simulink model "modelo"  (R2021b)
settings: Solver=VariableStepAuto  StartTime=0.0  StopTime=10.0  RelTol=1e-3
settings Model: Creator=iguil  LastModifiedBy=David

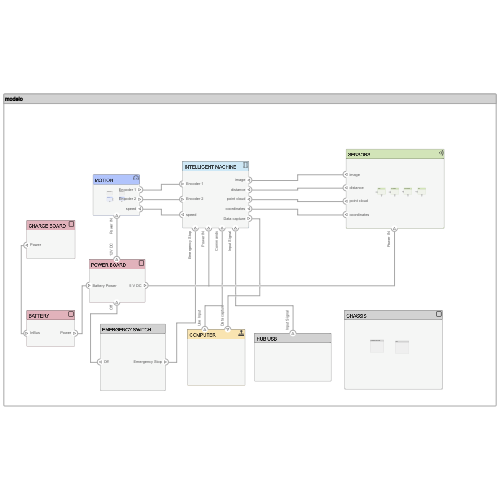
[thumbnail: Simulink's stored preview of the top-level diagram]
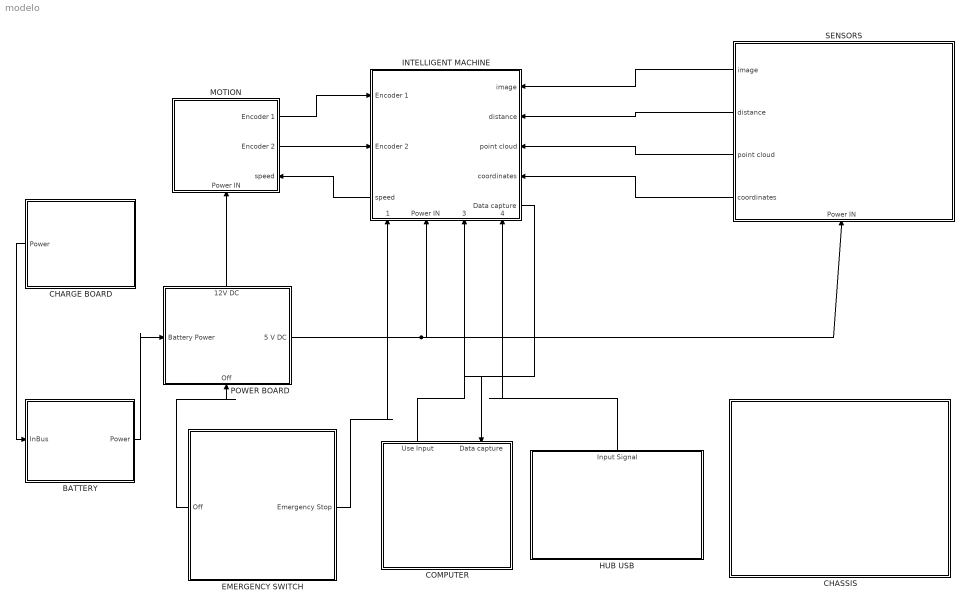
== system modelo ==
  BATTERY : Subsystem
      settings: PortSchema="{\"entries\":[{\"content\":{\"headerSize\":26,\"margin\":15,\"minimumSpacing\":25,\"sides\":[{\"content\":{\"connectorIds\":[\"In1\"]},\"type\":\"ConnectorPlacement.EquallySpacedRectSide\",\"uuid\":\"78ec9596-c19b-4a19-90cc-d79d904dcecb\"},{\"content\":{\"connectorIds\":[\"Out1\"],\"side\":\"RIGHT\"},\"type\":\"ConnectorPlacement.EquallySpacedRectSide\",\"uuid\":\"e50c32f8-61a1-4c3e-810e-7c092ec61b9d\"},{\"content\":{\"connectorIds\":[],\"side\":\"TOP\"},\"type\":\"ConnectorPlacement.EquallySpacedRectSide\",\"uuid\":\"dd5589de-c446-44bc-b6c3-43d178c94f81\"}]},\"type\":\"ConnectorPlacement.EquallySpacedConnector\",\"uuid\":\"1e9f716a-1f22-4423-b94e-8264810d47f5\"}],\"packageUris\":[\"http://schema.mathworks.com/mf0/Connector/R2020b\"],\"version\":\"1.0\"}"
  CHARGE BOARD : Subsystem
      settings: PortSchema="{\"entries\":[{\"content\":{\"headerSize\":26,\"margin\":15,\"minimumSpacing\":25,\"sides\":[{\"content\":{\"connectorIds\":[\"Out1\"]},\"type\":\"ConnectorPlacement.EquallySpacedRectSide\",\"uuid\":\"78ec9596-c19b-4a19-90cc-d79d904dcecb\"},{\"content\":{\"connectorIds\":[],\"side\":\"RIGHT\"},\"type\":\"ConnectorPlacement.EquallySpacedRectSide\",\"uuid\":\"e50c32f8-61a1-4c3e-810e-7c092ec61b9d\"},{\"content\":{\"connectorIds\":[],\"side\":\"TOP\"},\"type\":\"ConnectorPlacement.EquallySpacedRectSide\",\"uuid\":\"dd5589de-c446-44bc-b6c3-43d178c94f81\"},{\"content\":{\"connectorIds\":[],\"side\":\"BOTTOM\"},\"type\":\"ConnectorPlacement.EquallySpacedRectSide\",\"uuid\":\"27b2c156-9ba5-4a85-9e63-882de663826b\"}]},\"type\":\"ConnectorPlacement.EquallySpacedConnector\",\"uuid\":\"1e9f716a-1f22-4423-b94e-8264810d47f5\"}],\"packageUris\":[\"http://schema.mathworks.com/mf0/Connector/R2020b\"],\"version\":\"1.0\"}"
  CHASSIS : Subsystem
      settings: PortSchema="{\"entries\":[{\"content\":{\"headerSize\":26,\"margin\":15,\"minimumSpacing\":25,\"sides\":[{\"content\":{\"connectorIds\":[]},\"type\":\"ConnectorPlacement.EquallySpacedRectSide\",\"uuid\":\"78ec9596-c19b-4a19-90cc-d79d904dcecb\"},{\"content\":{\"connectorIds\":[],\"side\":\"RIGHT\"},\"type\":\"ConnectorPlacement.EquallySpacedRectSide\",\"uuid\":\"e50c32f8-61a1-4c3e-810e-7c092ec61b9d\"},{\"content\":{\"connectorIds\":[],\"side\":\"TOP\"},\"type\":\"ConnectorPlacement.EquallySpacedRectSide\",\"uuid\":\"dd5589de-c446-44bc-b6c3-43d178c94f81\"}]},\"type\":\"ConnectorPlacement.EquallySpacedConnector\",\"uuid\":\"1e9f716a-1f22-4423-b94e-8264810d47f5\"}],\"packageUris\":[\"http://schema.mathworks.com/mf0/Connector/R2020b\"],\"version\":\"1.0\"}"
  COMPUTER : Subsystem
      settings: PortSchema="{\"entries\":[{\"content\":{\"headerSize\":26,\"margin\":15,\"minimumSpacing\":25,\"sides\":[{\"content\":{\"connectorIds\":[]},\"type\":\"ConnectorPlacement.EquallySpacedRectSide\",\"uuid\":\"78ec9596-c19b-4a19-90cc-d79d904dcecb\"},{\"content\":{\"connectorIds\":[],\"side\":\"RIGHT\"},\"type\":\"ConnectorPlacement.EquallySpacedRectSide\",\"uuid\":\"e50c32f8-61a1-4c3e-810e-7c092ec61b9d\"},{\"content\":{\"connectorIds\":[\"Out1\",\"In1\"],\"side\":\"TOP\"},\"type\":\"ConnectorPlacement.EquallySpacedRectSide\",\"uuid\":\"dd5589de-c446-44bc-b6c3-43d178c94f81\"}]},\"type\":\"ConnectorPlacement.EquallySpacedConnector\",\"uuid\":\"1e9f716a-1f22-4423-b94e-8264810d47f5\"}],\"packageUris\":[\"http://schema.mathworks.com/mf0/Connector/R2020b\"],\"version\":\"1.0\"}"
  EMERGENCY SWITCH : Subsystem
      settings: PortSchema="{\"entries\":[{\"content\":{\"headerSize\":26,\"margin\":15,\"minimumSpacing\":25,\"sides\":[{\"content\":{\"connectorIds\":[\"Out1\"]},\"type\":\"ConnectorPlacement.EquallySpacedRectSide\",\"uuid\":\"b3e59be9-c011-4959-aae7-924c85fec7bb\"},{\"content\":{\"connectorIds\":[\"Out2\"],\"side\":\"RIGHT\"},\"type\":\"ConnectorPlacement.EquallySpacedRectSide\",\"uuid\":\"1b4348cb-da5a-4ff5-ba36-0dfb750bb370\"},{\"content\":{\"connectorIds\":[],\"side\":\"TOP\"},\"type\":\"ConnectorPlacement.EquallySpacedRectSide\",\"uuid\":\"b059a036-e728-494e-885b-23330087d2f9\"},{\"content\":{\"connectorIds\":[],\"side\":\"BOTTOM\"},\"type\":\"ConnectorPlacement.EquallySpacedRectSide\",\"uuid\":\"1d25428c-8dbd-4571-8b86-c34d6589503b\"}]},\"type\":\"ConnectorPlacement.EquallySpacedConnector\",\"uuid\":\"d162fe16-67ad-48b8-8b82-50f283e6c9c2\"}],\"packageUris\":[\"http://schema.mathworks.com/mf0/Connector/R2020b\"],\"version\":\"1.0\"}"
  HUB USB : Subsystem
      settings: PortSchema="{\"entries\":[{\"content\":{\"headerSize\":26,\"margin\":15,\"minimumSpacing\":25,\"sides\":[{\"content\":{\"connectorIds\":[]},\"type\":\"ConnectorPlacement.EquallySpacedRectSide\",\"uuid\":\"78ec9596-c19b-4a19-90cc-d79d904dcecb\"},{\"content\":{\"connectorIds\":[],\"side\":\"RIGHT\"},\"type\":\"ConnectorPlacement.EquallySpacedRectSide\",\"uuid\":\"e50c32f8-61a1-4c3e-810e-7c092ec61b9d\"},{\"content\":{\"connectorIds\":[\"Out1\"],\"side\":\"TOP\"},\"type\":\"ConnectorPlacement.EquallySpacedRectSide\",\"uuid\":\"dd5589de-c446-44bc-b6c3-43d178c94f81\"}]},\"type\":\"ConnectorPlacement.EquallySpacedConnector\",\"uuid\":\"1e9f716a-1f22-4423-b94e-8264810d47f5\"}],\"packageUris\":[\"http://schema.mathworks.com/mf0/Connector/R2020b\"],\"version\":\"1.0\"}"
  INTELLIGENT MACHINE : Subsystem
      settings: PortSchema="{\"entries\":[{\"content\":{\"headerSize\":26,\"margin\":15,\"minimumSpacing\":25,\"sides\":[{\"content\":{\"connectorIds\":[\"In8\",\"In9\",\"Out2\"]},\"type\":\"ConnectorPlacement.EquallySpacedRectSide\",\"uuid\":\"b3e59be9-c011-4959-aae7-924c85fec7bb\"},{\"content\":{\"connectorIds\":[\"In2\",\"In5\",\"In6\",\"In7\",\"Out1\"],\"side\":\"RIGHT\"},\"type\":\"ConnectorPlacement.EquallySpacedRectSide\",\"uuid\":\"1b4348cb-da5a-4ff5-ba36-0dfb750bb370\"},{\"content\":{\"connectorIds\":[],\"side\":\"TOP\"},\"type\":\"ConnectorPlacement.EquallySpacedRectSide\",\"uuid\":\"b059a036-e728-494e-885b-23330087d2f9\"},{\"content\":{\"connectorIds\":[\"In1\",\"In10\",\"In3\",\"In4\"],\"side\":\"BOTTOM\"},\"type\":\"ConnectorPlacement.EquallySpacedRectSide\",\"uuid\":\"1d25428c-8dbd-4571-8b86-c34d6589503b\"}]},\"type\":\"ConnectorPlacement.EquallySpacedConnector\",\"uuid\":\"d162fe16-67ad-48b8-8b82-50f283e6c9c2\"}],\"packageUris\":[\"http://schema.mathworks.com/mf0/Connector/R2020b\"],\"version\":\"1.0\"}"
  MOTION : Subsystem
      settings: PortSchema="{\"entries\":[{\"content\":{\"headerSize\":26,\"margin\":15,\"minimumSpacing\":25,\"sides\":[{\"content\":{\"connectorIds\":[]},\"type\":\"ConnectorPlacement.EquallySpacedRectSide\",\"uuid\":\"baaf5190-1ffc-4710-9f12-f4ddd1b73331\"},{\"content\":{\"connectorIds\":[\"Out1\",\"Out2\",\"In1\"],\"side\":\"RIGHT\"},\"type\":\"ConnectorPlacement.EquallySpacedRectSide\",\"uuid\":\"f5fb468f-cc96-476c-be3d-ed2ea869153e\"},{\"content\":{\"connectorIds\":[],\"side\":\"TOP\"},\"type\":\"ConnectorPlacement.EquallySpacedRectSide\",\"uuid\":\"45f5cb0d-60bf-4943-bb4c-a92d305a6805\"},{\"content\":{\"connectorIds\":[\"In2\"],\"side\":\"BOTTOM\"},\"type\":\"ConnectorPlacement.EquallySpacedRectSide\",\"uuid\":\"76d560be-4d0b-4cec-a6c5-6844847a893b\"}]},\"type\":\"ConnectorPlacement.EquallySpacedConnector\",\"uuid\":\"99c88219-ed2b-4820-8e38-f370b921e53e\"}],\"packageUris\":[\"http://schema.mathworks.com/mf0/Connector/R2020b\"],\"version\":\"1.0\"}"
  POWER BOARD : Subsystem
      settings: PortSchema="{\"entries\":[{\"content\":{\"headerSize\":26,\"margin\":15,\"minimumSpacing\":25,\"sides\":[{\"content\":{\"connectorIds\":[\"In2\"]},\"type\":\"ConnectorPlacement.EquallySpacedRectSide\",\"uuid\":\"baaf5190-1ffc-4710-9f12-f4ddd1b73331\"},{\"content\":{\"connectorIds\":[\"Out1\"],\"side\":\"RIGHT\"},\"type\":\"ConnectorPlacement.EquallySpacedRectSide\",\"uuid\":\"f5fb468f-cc96-476c-be3d-ed2ea869153e\"},{\"content\":{\"connectorIds\":[\"Out2\"],\"side\":\"TOP\"},\"type\":\"ConnectorPlacement.EquallySpacedRectSide\",\"uuid\":\"45f5cb0d-60bf-4943-bb4c-a92d305a6805\"},{\"content\":{\"connectorIds\":[\"In1\"],\"side\":\"BOTTOM\"},\"type\":\"ConnectorPlacement.EquallySpacedRectSide\",\"uuid\":\"91e60d79-0ecf-4e13-8fec-0c93feeae387\"}]},\"type\":\"ConnectorPlacement.EquallySpacedConnector\",\"uuid\":\"99c88219-ed2b-4820-8e38-f370b921e53e\"}],\"packageUris\":[\"http://schema.mathworks.com/mf0/Connector/R2020b\"],\"version\":\"1.0\"}"
  SENSORS : Subsystem
      settings: PortSchema="{\"entries\":[{\"content\":{\"headerSize\":26,\"margin\":15,\"minimumSpacing\":25,\"sides\":[{\"content\":{\"connectorIds\":[\"Out1\",\"Out2\",\"Out3\",\"Out4\"]},\"type\":\"ConnectorPlacement.EquallySpacedRectSide\",\"uuid\":\"b3e59be9-c011-4959-aae7-924c85fec7bb\"},{\"content\":{\"connectorIds\":[],\"side\":\"RIGHT\"},\"type\":\"ConnectorPlacement.EquallySpacedRectSide\",\"uuid\":\"1b4348cb-da5a-4ff5-ba36-0dfb750bb370\"},{\"content\":{\"connectorIds\":[],\"side\":\"TOP\"},\"type\":\"ConnectorPlacement.EquallySpacedRectSide\",\"uuid\":\"b059a036-e728-494e-885b-23330087d2f9\"},{\"content\":{\"connectorIds\":[\"In1\"],\"side\":\"BOTTOM\"},\"type\":\"ConnectorPlacement.EquallySpacedRectSide\",\"uuid\":\"ce80a790-94bd-4cfd-86e3-323fc0e3e1be\"}]},\"type\":\"ConnectorPlacement.EquallySpacedConnector\",\"uuid\":\"d162fe16-67ad-48b8-8b82-50f283e6c9c2\"}],\"packageUris\":[\"http://schema.mathworks.com/mf0/Connector/R2020b\"],\"version\":\"1.0\"}"
  wires:
  POWER BOARD/2(12V DC) -> MOTION/2(Power IN)
  INTELLIGENT MACHINE/2(speed) -> MOTION/1(speed)
  MOTION/1(Encoder 1) -> INTELLIGENT MACHINE/8(Encoder 1)
  MOTION/2(Encoder 2) -> INTELLIGENT MACHINE/9(Encoder 2)
  SENSORS/2(distance) -> INTELLIGENT MACHINE/5(distance)
  SENSORS/3(point cloud) -> INTELLIGENT MACHINE/6(point cloud)
  BATTERY/1(Power) -> POWER BOARD/2(Battery Power)
  CHARGE BOARD/1(Power) -> BATTERY/1(InBus)
  POWER BOARD/1(5 V DC) -> SENSORS/1(Power IN), INTELLIGENT MACHINE/10(Power IN)
  COMPUTER/1(Use Input) -> INTELLIGENT MACHINE/3(Commands)
  EMERGENCY SWITCH/2(Emergency Stop) -> INTELLIGENT MACHINE/1(Emergency Stop)
  EMERGENCY SWITCH/1(Off) -> POWER BOARD/1(Off)
  HUB USB/1(Input Signal) -> INTELLIGENT MACHINE/4(Input Signal)
  INTELLIGENT MACHINE/1(Data capture) -> COMPUTER/1(Data capture)
  SENSORS/4(coordinates) -> INTELLIGENT MACHINE/7(coordinates)
  SENSORS/1(image) -> INTELLIGENT MACHINE/2(image)

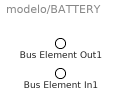
== system modelo/BATTERY ==
  Bus Element In1 : Inport  PortName=InBus
  Bus Element Out1 : Outport  PortName=Power

== system modelo/CHARGE BOARD ==
  Bus Element Out2 : Outport  PortName=Power

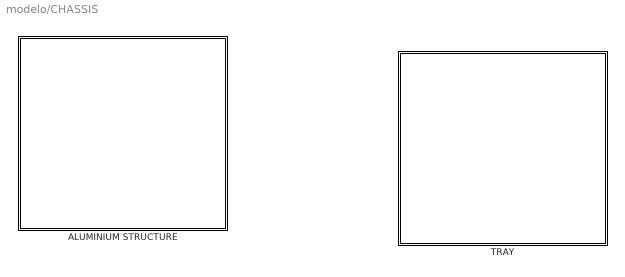
== system modelo/CHASSIS ==
  ALUMINIUM STRUCTURE : Subsystem
      settings: PortSchema="{\"entries\":[{\"content\":{\"headerSize\":26,\"margin\":15,\"minimumSpacing\":25,\"sides\":[{\"content\":{\"connectorIds\":[]},\"type\":\"ConnectorPlacement.EquallySpacedRectSide\",\"uuid\":\"78ec9596-c19b-4a19-90cc-d79d904dcecb\"},{\"content\":{\"connectorIds\":[],\"side\":\"RIGHT\"},\"type\":\"ConnectorPlacement.EquallySpacedRectSide\",\"uuid\":\"e50c32f8-61a1-4c3e-810e-7c092ec61b9d\"},{\"content\":{\"connectorIds\":[],\"side\":\"TOP\"},\"type\":\"ConnectorPlacement.EquallySpacedRectSide\",\"uuid\":\"dd5589de-c446-44bc-b6c3-43d178c94f81\"}]},\"type\":\"ConnectorPlacement.EquallySpacedConnector\",\"uuid\":\"1e9f716a-1f22-4423-b94e-8264810d47f5\"}],\"packageUris\":[\"http://schema.mathworks.com/mf0/Connector/R2020b\"],\"version\":\"1.0\"}"
  TRAY : Subsystem
      settings: PortSchema="{\"entries\":[{\"content\":{\"headerSize\":26,\"margin\":15,\"minimumSpacing\":25,\"sides\":[{\"content\":{\"connectorIds\":[]},\"type\":\"ConnectorPlacement.EquallySpacedRectSide\",\"uuid\":\"78ec9596-c19b-4a19-90cc-d79d904dcecb\"},{\"content\":{\"connectorIds\":[],\"side\":\"RIGHT\"},\"type\":\"ConnectorPlacement.EquallySpacedRectSide\",\"uuid\":\"e50c32f8-61a1-4c3e-810e-7c092ec61b9d\"},{\"content\":{\"connectorIds\":[],\"side\":\"TOP\"},\"type\":\"ConnectorPlacement.EquallySpacedRectSide\",\"uuid\":\"dd5589de-c446-44bc-b6c3-43d178c94f81\"}]},\"type\":\"ConnectorPlacement.EquallySpacedConnector\",\"uuid\":\"1e9f716a-1f22-4423-b94e-8264810d47f5\"}],\"packageUris\":[\"http://schema.mathworks.com/mf0/Connector/R2020b\"],\"version\":\"1.0\"}"

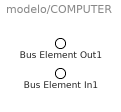
== system modelo/COMPUTER ==
  Bus Element In1 : Inport  PortName=Data capture
  Bus Element Out1 : Outport  PortName=Use Input

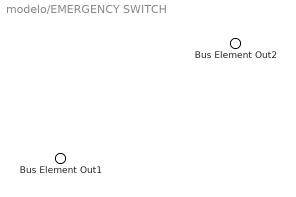
== system modelo/EMERGENCY SWITCH ==
  Bus Element Out2 : Outport  PortName=Off
  Bus Element Out1 : Outport  Port=2  PortName=Emergency Stop

== system modelo/HUB USB ==
  Bus Element Out1 : Outport  PortName=Input Signal

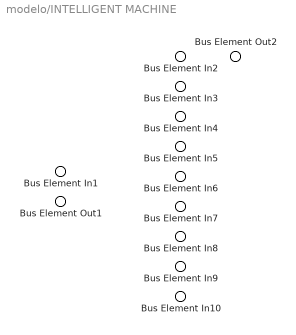
== system modelo/INTELLIGENT MACHINE ==
  Bus Element In9 : Inport  PortName=Emergency Stop
  Bus Element In5 : Inport  Port=2  PortName=image
  Bus Element In8 : Inport  Port=3  PortName=Commands
  Bus Element In10 : Inport  Port=4  PortName=Input Signal
  Bus Element In6 : Inport  Port=5  PortName=distance
  Bus Element In7 : Inport  Port=6  PortName=point cloud
  Bus Element In4 : Inport  Port=7  PortName=coordinates
  Bus Element In2 : Inport  Port=8  PortName=Encoder 1
  Bus Element In3 : Inport  Port=9  PortName=Encoder 2
  Bus Element In1 : Inport  Port=10  PortName=Power IN
  Bus Element Out2 : Outport  PortName=Data capture
  Bus Element Out1 : Outport  Port=2  PortName=speed

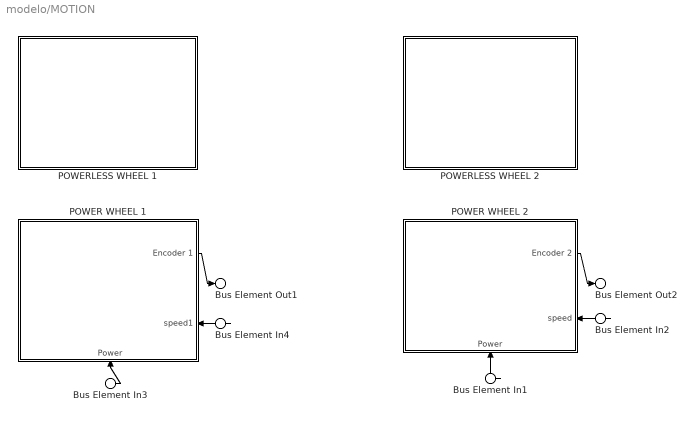
== system modelo/MOTION ==
  Bus Element In4 : Inport  PortName=speed  Element=1
  Bus Element In2 : Inport  PortName=speed  Element=2
  Bus Element In1 : Inport  Port=2  PortName=Power IN
  Bus Element In3 : Inport  Port=2  PortName=Power IN
  POWER WHEEL 1 : Subsystem
      settings: PortSchema="{\"entries\":[{\"content\":{\"headerSize\":26,\"margin\":15,\"minimumSpacing\":25,\"sides\":[{\"content\":{\"connectorIds\":[]},\"type\":\"ConnectorPlacement.EquallySpacedRectSide\",\"uuid\":\"b3e59be9-c011-4959-aae7-924c85fec7bb\"},{\"content\":{\"connectorIds\":[\"Out1\",\"In1\"],\"side\":\"RIGHT\"},\"type\":\"ConnectorPlacement.EquallySpacedRectSide\",\"uuid\":\"1b4348cb-da5a-4ff5-ba36-0dfb750bb370\"},{\"content\":{\"connectorIds\":[],\"side\":\"TOP\"},\"type\":\"ConnectorPlacement.EquallySpacedRectSide\",\"uuid\":\"b059a036-e728-494e-885b-23330087d2f9\"},{\"content\":{\"connectorIds\":[\"In2\"],\"side\":\"BOTTOM\"},\"type\":\"ConnectorPlacement.EquallySpacedRectSide\",\"uuid\":\"41224f02-e1ea-44d3-a03d-a24ecad52065\"}]},\"type\":\"ConnectorPlacement.EquallySpacedConnector\",\"uuid\":\"d162fe16-67ad-48b8-8b82-50f283e6c9c2\"}],\"packageUris\":[\"http://schema.mathworks.com/mf0/Connector/R2020b\"],\"version\":\"1.0\"}"
  POWER WHEEL 2 : Subsystem
      settings: PortSchema="{\"entries\":[{\"content\":{\"headerSize\":26,\"margin\":15,\"minimumSpacing\":25,\"sides\":[{\"content\":{\"connectorIds\":[]},\"type\":\"ConnectorPlacement.EquallySpacedRectSide\",\"uuid\":\"b3e59be9-c011-4959-aae7-924c85fec7bb\"},{\"content\":{\"connectorIds\":[\"Out1\",\"In2\"],\"side\":\"RIGHT\"},\"type\":\"ConnectorPlacement.EquallySpacedRectSide\",\"uuid\":\"1b4348cb-da5a-4ff5-ba36-0dfb750bb370\"},{\"content\":{\"connectorIds\":[],\"side\":\"TOP\"},\"type\":\"ConnectorPlacement.EquallySpacedRectSide\",\"uuid\":\"b059a036-e728-494e-885b-23330087d2f9\"},{\"content\":{\"connectorIds\":[\"In1\"],\"side\":\"BOTTOM\"},\"type\":\"ConnectorPlacement.EquallySpacedRectSide\",\"uuid\":\"9f493690-9325-494d-a5fd-d72c959f3b1f\"}]},\"type\":\"ConnectorPlacement.EquallySpacedConnector\",\"uuid\":\"d162fe16-67ad-48b8-8b82-50f283e6c9c2\"}],\"packageUris\":[\"http://schema.mathworks.com/mf0/Connector/R2020b\"],\"version\":\"1.0\"}"
  POWERLESS WHEEL 1 : Subsystem
      settings: PortSchema="{\"entries\":[{\"content\":{\"headerSize\":26,\"margin\":15,\"minimumSpacing\":25,\"sides\":[{\"content\":{\"connectorIds\":[]},\"type\":\"ConnectorPlacement.EquallySpacedRectSide\",\"uuid\":\"78ec9596-c19b-4a19-90cc-d79d904dcecb\"},{\"content\":{\"connectorIds\":[],\"side\":\"RIGHT\"},\"type\":\"ConnectorPlacement.EquallySpacedRectSide\",\"uuid\":\"e50c32f8-61a1-4c3e-810e-7c092ec61b9d\"},{\"content\":{\"connectorIds\":[],\"side\":\"TOP\"},\"type\":\"ConnectorPlacement.EquallySpacedRectSide\",\"uuid\":\"dd5589de-c446-44bc-b6c3-43d178c94f81\"},{\"content\":{\"connectorIds\":[],\"side\":\"BOTTOM\"},\"type\":\"ConnectorPlacement.EquallySpacedRectSide\",\"uuid\":\"3781c71a-b076-4a7f-bb10-0f0bb4f302b4\"}]},\"type\":\"ConnectorPlacement.EquallySpacedConnector\",\"uuid\":\"1e9f716a-1f22-4423-b94e-8264810d47f5\"}],\"packageUris\":[\"http://schema.mathworks.com/mf0/Connector/R2020b\"],\"version\":\"1.0\"}"
  POWERLESS WHEEL 2 : Subsystem
      settings: PortSchema="{\"entries\":[{\"content\":{\"headerSize\":26,\"margin\":15,\"minimumSpacing\":25,\"sides\":[{\"content\":{\"connectorIds\":[]},\"type\":\"ConnectorPlacement.EquallySpacedRectSide\",\"uuid\":\"78ec9596-c19b-4a19-90cc-d79d904dcecb\"},{\"content\":{\"connectorIds\":[],\"side\":\"RIGHT\"},\"type\":\"ConnectorPlacement.EquallySpacedRectSide\",\"uuid\":\"e50c32f8-61a1-4c3e-810e-7c092ec61b9d\"},{\"content\":{\"connectorIds\":[],\"side\":\"TOP\"},\"type\":\"ConnectorPlacement.EquallySpacedRectSide\",\"uuid\":\"dd5589de-c446-44bc-b6c3-43d178c94f81\"}]},\"type\":\"ConnectorPlacement.EquallySpacedConnector\",\"uuid\":\"1e9f716a-1f22-4423-b94e-8264810d47f5\"}],\"packageUris\":[\"http://schema.mathworks.com/mf0/Connector/R2020b\"],\"version\":\"1.0\"}"
  Bus Element Out1 : Outport  PortName=Encoder 1
  Bus Element Out2 : Outport  Port=2  PortName=Encoder 2
  wires:
  Bus Element In2/1 -> POWER WHEEL 2/2(speed)
  Bus Element In1/1 -> POWER WHEEL 2/1(Power)
  Bus Element In3/1 -> POWER WHEEL 1/2(Power)
  Bus Element In4/1 -> POWER WHEEL 1/1(speed1)
  POWER WHEEL 1/1(Encoder 1) -> Bus Element Out1/1
  POWER WHEEL 2/1(Encoder 2) -> Bus Element Out2/1

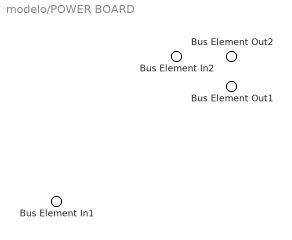
== system modelo/POWER BOARD ==
  Bus Element In2 : Inport  PortName=Off
  Bus Element In1 : Inport  Port=2  PortName=Battery Power
  Bus Element Out1 : Outport  PortName=5 V DC
  Bus Element Out2 : Outport  Port=2  PortName=12V DC

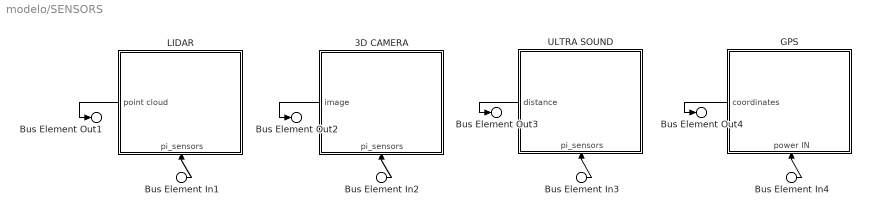
== system modelo/SENSORS ==
  Bus Element In{1..4} (4 alike) : Inport  PortName=Power IN
  3D CAMERA : Subsystem
      settings: PortSchema="{\"entries\":[{\"content\":{\"headerSize\":26,\"margin\":15,\"minimumSpacing\":25,\"sides\":[{\"content\":{\"connectorIds\":[\"Out1\"]},\"type\":\"ConnectorPlacement.EquallySpacedRectSide\",\"uuid\":\"b3e59be9-c011-4959-aae7-924c85fec7bb\"},{\"content\":{\"connectorIds\":[],\"side\":\"RIGHT\"},\"type\":\"ConnectorPlacement.EquallySpacedRectSide\",\"uuid\":\"1b4348cb-da5a-4ff5-ba36-0dfb750bb370\"},{\"content\":{\"connectorIds\":[],\"side\":\"TOP\"},\"type\":\"ConnectorPlacement.EquallySpacedRectSide\",\"uuid\":\"b059a036-e728-494e-885b-23330087d2f9\"},{\"content\":{\"connectorIds\":[\"In1\"],\"side\":\"BOTTOM\"},\"type\":\"ConnectorPlacement.EquallySpacedRectSide\",\"uuid\":\"029e8ecc-94c5-4d9d-93c4-0362b1480c7f\"}]},\"type\":\"ConnectorPlacement.EquallySpacedConnector\",\"uuid\":\"d162fe16-67ad-48b8-8b82-50f283e6c9c2\"}],\"packageUris\":[\"http://schema.mathworks.com/mf0/Connector/R2020b\"],\"version\":\"1.0\"}"
  GPS : Subsystem
      settings: PortSchema="{\"entries\":[{\"content\":{\"headerSize\":26,\"margin\":15,\"minimumSpacing\":25,\"sides\":[{\"content\":{\"connectorIds\":[\"Out1\"]},\"type\":\"ConnectorPlacement.EquallySpacedRectSide\",\"uuid\":\"b3e59be9-c011-4959-aae7-924c85fec7bb\"},{\"content\":{\"connectorIds\":[],\"side\":\"RIGHT\"},\"type\":\"ConnectorPlacement.EquallySpacedRectSide\",\"uuid\":\"1b4348cb-da5a-4ff5-ba36-0dfb750bb370\"},{\"content\":{\"connectorIds\":[],\"side\":\"TOP\"},\"type\":\"ConnectorPlacement.EquallySpacedRectSide\",\"uuid\":\"b059a036-e728-494e-885b-23330087d2f9\"},{\"content\":{\"connectorIds\":[\"In1\"],\"side\":\"BOTTOM\"},\"type\":\"ConnectorPlacement.EquallySpacedRectSide\",\"uuid\":\"29b5170b-1118-48f5-8bd8-b1ab2474e927\"}]},\"type\":\"ConnectorPlacement.EquallySpacedConnector\",\"uuid\":\"d162fe16-67ad-48b8-8b82-50f283e6c9c2\"}],\"packageUris\":[\"http://schema.mathworks.com/mf0/Connector/R2020b\"],\"version\":\"1.0\"}"
  LIDAR : Subsystem
      settings: PortSchema="{\"entries\":[{\"content\":{\"headerSize\":26,\"margin\":15,\"minimumSpacing\":25,\"sides\":[{\"content\":{\"connectorIds\":[\"Out1\"]},\"type\":\"ConnectorPlacement.EquallySpacedRectSide\",\"uuid\":\"b3e59be9-c011-4959-aae7-924c85fec7bb\"},{\"content\":{\"connectorIds\":[],\"side\":\"RIGHT\"},\"type\":\"ConnectorPlacement.EquallySpacedRectSide\",\"uuid\":\"1b4348cb-da5a-4ff5-ba36-0dfb750bb370\"},{\"content\":{\"connectorIds\":[],\"side\":\"TOP\"},\"type\":\"ConnectorPlacement.EquallySpacedRectSide\",\"uuid\":\"b059a036-e728-494e-885b-23330087d2f9\"},{\"content\":{\"connectorIds\":[\"In1\"],\"side\":\"BOTTOM\"},\"type\":\"ConnectorPlacement.EquallySpacedRectSide\",\"uuid\":\"28209bda-55bc-46ff-b97e-b75cf1cdc03d\"}]},\"type\":\"ConnectorPlacement.EquallySpacedConnector\",\"uuid\":\"d162fe16-67ad-48b8-8b82-50f283e6c9c2\"}],\"packageUris\":[\"http://schema.mathworks.com/mf0/Connector/R2020b\"],\"version\":\"1.0\"}"
  ULTRA SOUND : Subsystem
      settings: PortSchema="{\"entries\":[{\"content\":{\"headerSize\":26,\"margin\":15,\"minimumSpacing\":25,\"sides\":[{\"content\":{\"connectorIds\":[\"Out1\"]},\"type\":\"ConnectorPlacement.EquallySpacedRectSide\",\"uuid\":\"b3e59be9-c011-4959-aae7-924c85fec7bb\"},{\"content\":{\"connectorIds\":[],\"side\":\"RIGHT\"},\"type\":\"ConnectorPlacement.EquallySpacedRectSide\",\"uuid\":\"1b4348cb-da5a-4ff5-ba36-0dfb750bb370\"},{\"content\":{\"connectorIds\":[],\"side\":\"TOP\"},\"type\":\"ConnectorPlacement.EquallySpacedRectSide\",\"uuid\":\"b059a036-e728-494e-885b-23330087d2f9\"},{\"content\":{\"connectorIds\":[\"In1\"],\"side\":\"BOTTOM\"},\"type\":\"ConnectorPlacement.EquallySpacedRectSide\",\"uuid\":\"8856fd7e-567b-4c50-a906-ab6a46c3f8be\"}]},\"type\":\"ConnectorPlacement.EquallySpacedConnector\",\"uuid\":\"d162fe16-67ad-48b8-8b82-50f283e6c9c2\"}],\"packageUris\":[\"http://schema.mathworks.com/mf0/Connector/R2020b\"],\"version\":\"1.0\"}"
  Bus Element Out2 : Outport  PortName=image
  Bus Element Out3 : Outport  Port=2  PortName=distance
  Bus Element Out1 : Outport  Port=3  PortName=point cloud
  Bus Element Out4 : Outport  Port=4  PortName=coordinates
  wires:
  Bus Element In1/1 -> LIDAR/1(pi_sensors)
  Bus Element In2/1 -> 3D CAMERA/1(pi_sensors)
  Bus Element In3/1 -> ULTRA SOUND/1(pi_sensors)
  LIDAR/1(point cloud) -> Bus Element Out1/1
  3D CAMERA/1(image) -> Bus Element Out2/1
  ULTRA SOUND/1(distance) -> Bus Element Out3/1
  Bus Element In4/1 -> GPS/1(power IN)
  GPS/1(coordinates) -> Bus Element Out4/1

== system modelo/CHASSIS/ALUMINIUM STRUCTURE ==

== system modelo/CHASSIS/TRAY ==

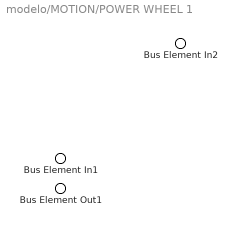
== system modelo/MOTION/POWER WHEEL 1 ==
  Bus Element In2 : Inport  PortName=speed1
  Bus Element In1 : Inport  Port=2  PortName=Power
  Bus Element Out1 : Outport  PortName=Encoder 1

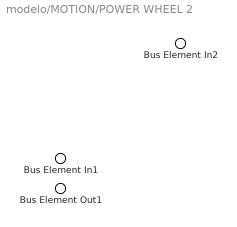
== system modelo/MOTION/POWER WHEEL 2 ==
  Bus Element In2 : Inport  PortName=Power
  Bus Element In1 : Inport  Port=2  PortName=speed
  Bus Element Out1 : Outport  PortName=Encoder 2

== system modelo/MOTION/POWERLESS WHEEL 1 ==

== system modelo/MOTION/POWERLESS WHEEL 2 ==

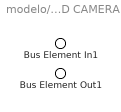
== system modelo/SENSORS/3D CAMERA ==
  Bus Element In1 : Inport  PortName=pi_sensors
  Bus Element Out1 : Outport  PortName=image

== system modelo/SENSORS/GPS ==
  Bus Element In1 : Inport  PortName=power IN
  Bus Element Out1 : Outport  PortName=coordinates

== system modelo/SENSORS/LIDAR ==
  Bus Element In1 : Inport  PortName=pi_sensors
  Bus Element Out1 : Outport  PortName=point cloud

== system modelo/SENSORS/ULTRA SOUND ==
  Bus Element In1 : Inport  PortName=pi_sensors
  Bus Element Out1 : Outport  PortName=distance
